simulink model "explicit_cruise_acc"  (R2021a)
settings: Solver=FixedStepAuto  StartTime=0.0  StopTime=inf  FixedStep=2.0  RelTol=1e-3
libraries: robotlib x10
settings Model: Creator=ivory  LastModifiedBy=sprinkle
settings SolverCC: AlgebraicLoopSolver=TrustRegion
settings OptimizationCC: EnhancedBackFolding=on  PassReuseOutputArgsAs=Individual arguments  ZeroExternalMemoryAtStartup=off  ZeroInternalMemoryAtStartup=off  MaxStackSize=64  OptimizeBlockOrder=speed  DifferentSizesBufferReuse=on  OptimizationCustomize=off  EfficientTunableParamExpr=on
settings DebuggingCC: ParameterTunabilityLossMsg=error  SFMachineParentedDataDiag=warning
settings HardwareCC: ProdBitPerPointer=32  ProdBitPerSizeT=32  ProdBitPerPtrDiffT=32  ProdLargestAtomicFloat=None  ProdIntDivRoundTo=Undefined  ProdEndianess=Unspecified  ProdWordSize=32  ProdHWDeviceType=Generic->Unspecified (assume 32-bit Generic)
settings SFSimCC: MATLABDynamicMemAlloc=off  SimTargetLang=C++
settings RTWCC: SystemTargetFile=ert.tlc  HardwareBoard=Robot Operating System (ROS)  TLCOptions="-aInlineSetEventsForThisBaseRateFcn=TLC_FALSE -aSuppressMultiTaskScheduler=TLC_FALSE  -aRateBasedStepFcn=0"  TemplateMakefile=ert_default_tmf  GenerateReport=on  Toolchain=Catkin  IncludeHyperlinkInReport=on  LaunchReport=on  TargetLang=C++  GenerateTraceInfo=on  GenerateTraceReport=on  GenerateTraceReportSl=on  GenerateTraceReportSf=on  GenerateTraceReportEml=on
settings CodeAppCC: ForceParamTrailComments=on  IgnoreCustomStorageClasses=off  OperatorAnnotations=on  SimulinkDataObjDesc=on  SFDataObjDesc=on  InsertBlockDesc=on
settings ERTTargetCC: SupportContinuousTime=on  SupportVariableSizeSignals=on

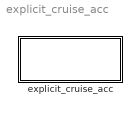
== system explicit_cruise_acc ==
  explicit_cruise_acc : Subsystem

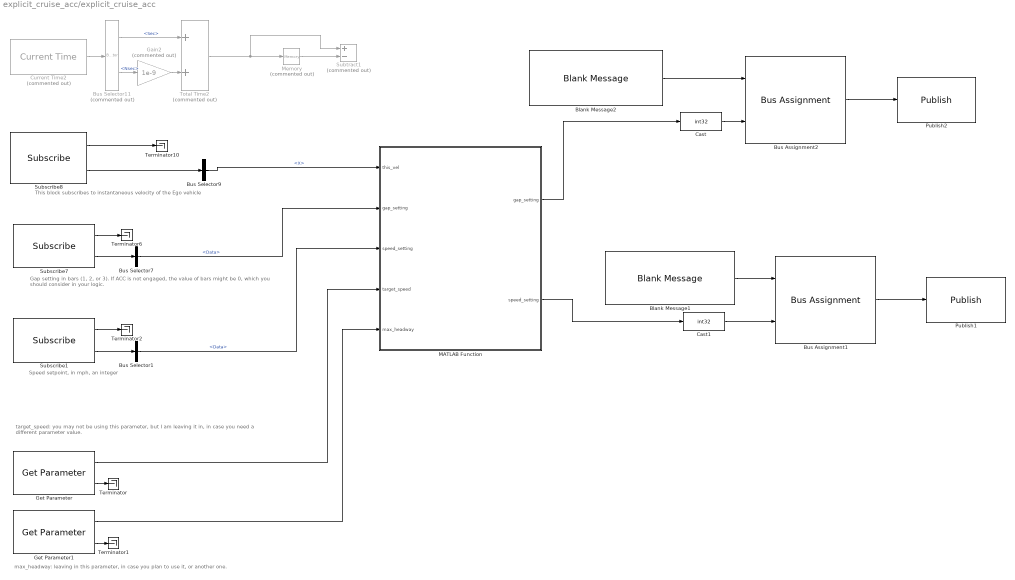
== system explicit_cruise_acc/explicit_cruise_acc ==
  note: Gap setting in bars (1, 2, or 3).
      | If ACC is not engaged, the value of bars might be 0, which you should consider in your logic.
  note: This block subscribes to
      | instantaneous velocity of the Ego vehicle
  note: Speed setpoint, in mph, an integer
  note: target_speed: you may not be using this parameter, but I am leaving it in, in case you need a different parameter value.
  note: max_headway: leaving in this parameter, in case you plan
      | to use it, or another one.
  Blank Message1 : robotlib/Blank Message  messageClass=Message  entityType=std_msgs/Int32  messageType=std_msgs/Int32  SampleTime=inf  legacyBusStruct=off
  Blank Message2 : robotlib/Blank Message  messageClass=Message  entityType=std_msgs/Int32  messageType=std_msgs/Int32  SampleTime=inf  legacyBusStruct=off
  Bus Assignment1 : BusAssignment  AssignedSignals=Data
  Bus Assignment2 : BusAssignment  AssignedSignals=Data
  Bus Selector1 : BusSelector  OutputSignals=Data
  Bus Selector11 : BusSelector  Commented=on  OutputSignals=Sec,Nsec
  Bus Selector7 : BusSelector  OutputSignals=Data
  Bus Selector9 : BusSelector  OutputSignals=Linear.X
  Cast : DataTypeConversion  OutDataTypeStr=int32
  Cast1 : DataTypeConversion  OutDataTypeStr=int32
  Current Time2 : robotlib/Current Time  Commented=on  OutputFormat=bus  SampleTime=-1  ModelName=microaccel
      settings: SourceProductBaseCode=RR
  Gain2 : Gain  Commented=on  Gain=1e-9
  Get Parameter : robotlib/Get Parameter  ParameterSource=Specify your own  ParameterName=target_speed  ParameterType=double  ParameterMaxArrayLength=16  ParameterInitialValue=25.0  SampleTime=-1  ShowErrorCodeOutput=on  ModelName=explicit_cruise_acc  BlockId=ParamGet_explicit_cruise_acc_655
      settings: SourceProductBaseCode=RR
  Get Parameter1 : robotlib/Get Parameter  ParameterSource=Specify your own  ParameterName=max_headway  ParameterType=double  ParameterMaxArrayLength=16  ParameterInitialValue=50.0  SampleTime=-1  ShowErrorCodeOutput=on  ModelName=explicit_cruise_acc  BlockId=ParamGet_explicit_cruise_acc_657
      settings: SourceProductBaseCode=RR
  MATLAB Function : MATLAB Function  TreatAsAtomicUnit=on
  Memory : Memory  Commented=on
  Publish1 : robotlib/Publish  topicSource=Specify your own  topic=speed_setting  messageType=std_msgs/Int32  legacyBusStruct=off  messageQueueLength=1
  Publish2 : robotlib/Publish  topicSource=Specify your own  topic=gap_setting  messageType=std_msgs/Int32  legacyBusStruct=off  messageQueueLength=1
  Subscribe1 : robotlib/Subscribe  topicSource=Specify your own  topic=speed_setting  messageType=std_msgs/Int32  SampleTime=-1  legacyBusStruct=off  messageQueueLength=1
  Subscribe7 : robotlib/Subscribe  topicSource=Specify your own  topic=gap_setting  messageType=std_msgs/Int32  SampleTime=-1  legacyBusStruct=off  messageQueueLength=1
  Subscribe8 : robotlib/Subscribe  topicSource=Specify your own  topic=vel  messageType=geometry_msgs/Twist  SampleTime=-1  legacyBusStruct=off  messageQueueLength=1
  Subtract1 : Sum  Commented=on  Inputs=+-
  Terminator{,1..2,6,10} (5 alike) : Terminator
  Total Time2 : Sum  Commented=on
  wires:
  Bus Selector11/1 -> Total Time2/1  "<Sec>"
  Gain2/1 -> Total Time2/2
  Bus Selector11/2 -> Gain2/1  "<Nsec>"
  Total Time2/1 -> Subtract1/1, Memory/1
  Current Time2/1 -> Bus Selector11/1
  Memory/1 -> Subtract1/2
  Subscribe8/2 -> Bus Selector9/1
  Subscribe8/1 -> Terminator10/1
  Bus Selector9/1 -> MATLAB Function/1(this_vel)  "<X>"
  Subscribe7/1 -> Terminator6/1
  Subscribe7/2 -> Bus Selector7/1
  Get Parameter/1 -> MATLAB Function/4(target_speed)
  Get Parameter/2 -> Terminator/1
  Get Parameter1/2 -> Terminator1/1
  Get Parameter1/1 -> MATLAB Function/5(max_headway)
  Bus Assignment2/1 -> Publish2/1
  Blank Message2/1 -> Bus Assignment2/1
  MATLAB Function/1(gap_setting) -> Cast/1
  Blank Message1/1 -> Bus Assignment1/1
  Bus Assignment1/1 -> Publish1/1
  Cast/1 -> Bus Assignment2/2
  Cast1/1 -> Bus Assignment1/2
  Subscribe1/1 -> Terminator2/1
  Subscribe1/2 -> Bus Selector1/1
  Bus Selector1/1 -> MATLAB Function/3("speed_setting ")  "<Data>"
  MATLAB Function/2(speed_setting) -> Cast1/1
  Bus Selector7/1 -> MATLAB Function/2("gap_setting ")  "<Data>"

== matlab function explicit_cruise_acc/MATLAB Function ==
  settings: updateMethod=DISCRETE
  data: this_vel input; gap_setting input; speed_setting input; gap_setting output; target_speed input; max_headway input; speed_setting output
function [gap_setting, speed_setting] =  get_acc_values(this_vel, gap_setting, speed_setting, target_speed, max_headway)
        %%"""See parent class."""
        % TODO (Amaury): replace with your controller's logic
        MPH_TO_MS = 0.44704;

end
